simulink model "rlCOMP"  (R2024b)
settings: Solver=FixedStepAuto  StartTime=0.0  StopTime=Tf  FixedStep=0.001  RelTol=1e-3
StartFcn:
  | %scopes= find_system(bdroot,'BlockType','Scope');
  | %for i = 1:length(scopes)
  | %set_param(scopes{i},'Open','on');
  | %end
values from neighbouring files (symbols this model uses):
  amax_ego = 0.4    [MADDPG4_1.m]    (also in MADDPG4__no_rules.m; RL_COMP.m)
  amin_ego = -0.5    [MADDPG4_1.m]    (also in MADDPG4__no_rules.m; RL_COMP.m)
  Cf = 19000    [MADDPG4_1.m]    (also in MADDPG4__no_rules.m; RL_COMP.m)
  Cr = 33000    [MADDPG4_1.m]    (also in MADDPG4__no_rules.m; RL_COMP.m)
  D_default = 1.5    [MADDPG4_1.m]    (also in MADDPG4__no_rules.m; RL_COMP.m)
  e1_initial = 0    [MADDPG4_1.m]    (also in MADDPG4__no_rules.m = -0.05; RL_COMP.m = -0.05)
  e2_initial = 0.26    [MADDPG4_1.m]    (also in MADDPG4__no_rules.m = 0.05; RL_COMP.m = 0.05)
  Iz = 2875    [MADDPG4_1.m]    (also in MADDPG4__no_rules.m; RL_COMP.m)
  lf = 1.4    [MADDPG4_1.m]    (also in MADDPG4__no_rules.m; RL_COMP.m)
  lr = 1.6    [MADDPG4_1.m]    (also in MADDPG4__no_rules.m; RL_COMP.m)
  m = 1600    [MADDPG4_1.m]    (also in MADDPG4__no_rules.m; RL_COMP.m)
  t_gap = 1.4    [MADDPG4_1.m]    (also in MADDPG4__no_rules.m; RL_COMP.m)
  target = 3    [MADDPG4_1.m]    (also in MADDPG4__no_rules.m; RL_COMP.m = 1)
  tau = 0.5    [MADDPG4_1.m]    (also in MADDPG4__no_rules.m; RL_COMP.m)
  Ts = 0.1    [MADDPG4_1.m]    (also in MADDPG4__no_rules.m; RL_COMP.m)
  umax_ego = 0.2618    [MADDPG4_1.m]    (also in MADDPG4__no_rules.m; RL_COMP.m)
  umin_ego = -0.2618    [MADDPG4_1.m]    (also in MADDPG4__no_rules.m; RL_COMP.m)
  v0_FV1 = 0.5    [MADDPG4_1.m]    (also in MADDPG4__no_rules.m; RL_COMP.m)
  v0_FV2 = 0.5    [MADDPG4_1.m]    (also in MADDPG4__no_rules.m; RL_COMP.m)
  v0_LV = 0.9    [MADDPG4_1.m]    (also in MADDPG4__no_rules.m; RL_COMP.m)
  v_set = 1.5    [MADDPG4_1.m]    (also in MADDPG4__no_rules.m; RL_COMP.m)
  x0_FV1 = 1.5    [MADDPG4_1.m]    (also in MADDPG4__no_rules.m; RL_COMP.m)
  x0_FV2 = 0    [MADDPG4_1.m]    (also in MADDPG4__no_rules.m; RL_COMP.m)
  x0_LV = 3    [MADDPG4_1.m]    (also in MADDPG4__no_rules.m; RL_COMP.m)
undefined symbols (not defined in the file or in its folder): DiscIntNeverNeededParam, Speed, SteeringAngle
libraries: simulink x19, rllib x4, robotlib x4, dspfdesign x2
(part 2 of 2)

== system rlCOMP/STEER3/Subsystem1 ==
  e1 : Inport
  e2 : Inport  Port=2
  e1dot : Inport  Port=3
  e2dot : Inport  Port=4
  steer2 : Inport  Port=5
  lat2 : Inport  Port=6
  yaw2 : Inport  Port=7
  Discrete-Time Integrator : DiscreteIntegrator  SampleTime=-1  ICPrevOutput=DiscIntNeverNeededParam  ICPrevScaledInput=DiscIntNeverNeededParam
  Discrete-Time Integrator1 : DiscreteIntegrator  SampleTime=-1  ICPrevOutput=DiscIntNeverNeededParam  ICPrevScaledInput=DiscIntNeverNeededParam
  Mux : Mux  Inputs=9
  obs : Outport  VectorParamsAs1DForOutWhenUnconnected=off
  wires:
  e1/1 -> Mux/2, Discrete-Time Integrator1/1
  Mux/1 -> obs/1
  Discrete-Time Integrator1/1 -> Mux/1  "integral_error"
  e2/1 -> Mux/4, Discrete-Time Integrator/1
  Discrete-Time Integrator/1 -> Mux/3  "integral_error"
  e1dot/1 -> Mux/5
  e2dot/1 -> Mux/6
  steer2/1 -> Mux/7
  lat2/1 -> Mux/8
  yaw2/1 -> Mux/9

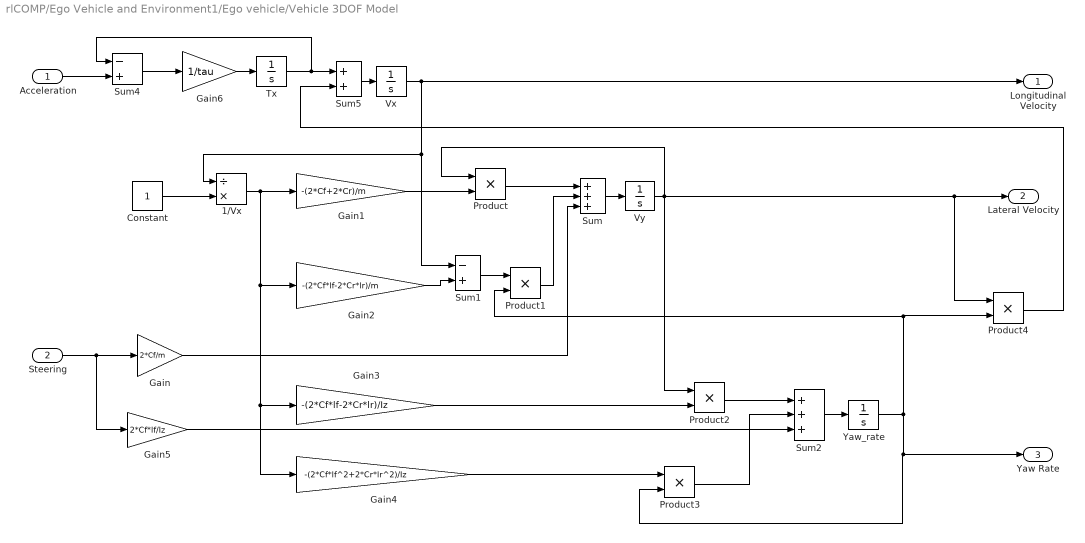
== system rlCOMP/Ego Vehicle and Environment1/Ego vehicle/Vehicle 3DOF Model ==
  Acceleration : Inport
  Steering : Inport  Port=2
  1/Vx : Product  Inputs=/*
  Constant : Constant
  Gain : Gain  Gain=2*Cf/m
  Gain1 : Gain  Gain=-(2*Cf+2*Cr)/m
  Gain2 : Gain  Gain=-(2*Cf*lf-2*Cr*lr)/m
  Gain3 : Gain  Gain=-(2*Cf*lf-2*Cr*lr)/Iz
  Gain4 : Gain  Gain=-(2*Cf*lf^2+2*Cr*lr^2)/Iz
  Gain5 : Gain  Gain=2*Cf*lf/Iz
  Gain6 : Gain  Gain=1/tau
  Product{,1..4} (5 alike) : Product
  Sum : Sum  Inputs=+++
  Sum1 : Sum  Inputs=-+
  Sum2 : Sum  Inputs=+++
  Sum4 : Sum  Inputs=-+
  Sum5 : Sum
  Tx : Integrator
  Vx : Integrator  InitialCondition=v0_FV2
  Vy : Integrator
  "Yaw_rate " : Integrator
  Longitudinal Velocity : Outport  VectorParamsAs1DForOutWhenUnconnected=off
  Lateral Velocity : Outport  Port=2  VectorParamsAs1DForOutWhenUnconnected=off
  Yaw Rate : Outport  Port=3  VectorParamsAs1DForOutWhenUnconnected=off
  wires:
  Vy/1 -> Product/1, Lateral Velocity/1, Product4/1, Product2/1
  Gain2/1 -> Sum1/2
  Product/1 -> Sum/1
  Tx/1 -> Sum5/1, Sum4/1
  Sum/1 -> Vy/1
  "Yaw_rate "/1 -> Yaw Rate/1, Product3/2, Product4/2, Product1/2
  1/Vx/1 -> Gain4/1, Gain3/1, Gain2/1, Gain1/1
  Vx/1 -> 1/Vx/1, Sum1/1, Longitudinal Velocity/1
  Product3/1 -> Sum2/2
  Steering/1 -> Gain/1, Gain5/1
  Acceleration/1 -> Sum4/2
  Sum1/1 -> Product1/1
  Gain/1 -> Sum/3
  Gain1/1 -> Product/2
  Gain6/1 -> Tx/1
  Product2/1 -> Sum2/1
  Sum5/1 -> Vx/1
  Constant/1 -> 1/Vx/2
  Product1/1 -> Sum/2
  Sum4/1 -> Gain6/1
  Gain4/1 -> Product3/1
  Product4/1 -> Sum5/2
  Gain3/1 -> Product2/2
  Gain5/1 -> Sum2/3
  Sum2/1 -> "Yaw_rate "/1

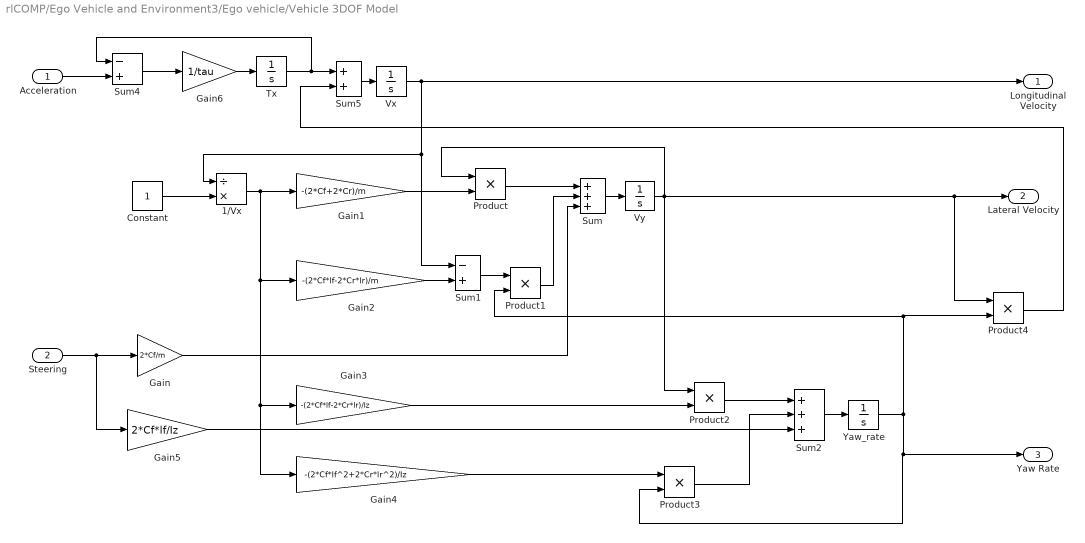
== system rlCOMP/Ego Vehicle and Environment3/Ego vehicle/Vehicle 3DOF Model ==
  Acceleration : Inport
  Steering : Inport  Port=2
  1/Vx : Product  Inputs=/*
  Constant : Constant
  Gain : Gain  Gain=2*Cf/m
  Gain1 : Gain  Gain=-(2*Cf+2*Cr)/m
  Gain2 : Gain  Gain=-(2*Cf*lf-2*Cr*lr)/m
  Gain3 : Gain  Gain=-(2*Cf*lf-2*Cr*lr)/Iz
  Gain4 : Gain  Gain=-(2*Cf*lf^2+2*Cr*lr^2)/Iz
  Gain5 : Gain  Gain=2*Cf*lf/Iz
  Gain6 : Gain  Gain=1/tau
  Product{,1..4} (5 alike) : Product
  Sum : Sum  Inputs=+++
  Sum1 : Sum  Inputs=-+
  Sum2 : Sum  Inputs=+++
  Sum4 : Sum  Inputs=-+
  Sum5 : Sum
  Tx : Integrator
  Vx : Integrator  InitialCondition=v0_FV1
  Vy : Integrator
  "Yaw_rate " : Integrator
  Longitudinal Velocity : Outport  VectorParamsAs1DForOutWhenUnconnected=off
  Lateral Velocity : Outport  Port=2  VectorParamsAs1DForOutWhenUnconnected=off
  Yaw Rate : Outport  Port=3  VectorParamsAs1DForOutWhenUnconnected=off
  wires:
  Vy/1 -> Product/1, Lateral Velocity/1, Product4/1, Product2/1
  Gain2/1 -> Sum1/2
  Product/1 -> Sum/1
  Tx/1 -> Sum5/1, Sum4/1
  Sum/1 -> Vy/1
  "Yaw_rate "/1 -> Yaw Rate/1, Product3/2, Product4/2, Product1/2
  1/Vx/1 -> Gain4/1, Gain3/1, Gain2/1, Gain1/1
  Vx/1 -> 1/Vx/1, Sum1/1, Longitudinal Velocity/1
  Product3/1 -> Sum2/2
  Steering/1 -> Gain/1, Gain5/1
  Acceleration/1 -> Sum4/2
  Sum1/1 -> Product1/1
  Gain/1 -> Sum/3
  Gain1/1 -> Product/2
  Gain6/1 -> Tx/1
  Product2/1 -> Sum2/1
  Sum5/1 -> Vx/1
  Constant/1 -> 1/Vx/2
  Product1/1 -> Sum/2
  Sum4/1 -> Gain6/1
  Gain4/1 -> Product3/1
  Product4/1 -> Sum5/2
  Gain3/1 -> Product2/2
  Gain5/1 -> Sum2/3
  Sum2/1 -> "Yaw_rate "/1

== system rlCOMP/Ego Vehicle and Environment3/Lead vehicle1/ramp1 ==
  note: 工况1：斜坡加速度
  Clock : Clock
  Constant1 : Constant  Value=20
  Constant2 : Constant  Value=40
  Ramp : simulink/Sources/Ramp  slope=0.001  start=0  InitialOutput=0
  Ramp1 : simulink/Sources/Ramp  slope=-0.001  start=20  InitialOutput=0.02
  Ramp2 : simulink/Sources/Ramp  slope=0  start=40  InitialOutput=0
  Relational Operator : RelationalOperator  Operator=<=  OutDataTypeStr=boolean  RndMeth=Simplest  InputSameDT=off
  Relational Operator1 : RelationalOperator  Operator=<=  OutDataTypeStr=boolean  RndMeth=Simplest  InputSameDT=off
  Switch : Switch  Criteria=u2 > Threshold  SaturateOnIntegerOverflow=off  InputSameDT=off
  Switch1 : Switch  Criteria=u2 > Threshold  SaturateOnIntegerOverflow=off  InputSameDT=off
  Out1 : Outport
  wires:
  Constant1/1 -> Relational Operator/2
  Ramp1/1 -> Switch1/1
  Relational Operator/1 -> Switch/2
  Switch1/1 -> Switch/3
  Relational Operator1/1 -> Switch1/2
  Clock/1 -> Relational Operator1/1, Relational Operator/1
  Ramp/1 -> Switch/1
  Constant2/1 -> Relational Operator1/2
  Ramp2/1 -> Switch1/3
  Switch/1 -> Out1/1

== system rlCOMP/Ego Vehicle and Environment3/Lead vehicle1/step1 ==
  note: 工况3：阶梯式加速-减速
  Add : Sum  Inputs=++++
  Step : Step  Time=5  After=0.2  SampleTime=0
  Step1 : Step  Time=8  After=-0.2  SampleTime=0
  Step2 : Step  Time=40  After=-0.2  SampleTime=0
  Step3 : Step  Time=43  After=0.2  SampleTime=0
  a_LV : Outport
  wires:
  Step2/1 -> Add/3
  Step3/1 -> Add/4
  Step/1 -> Add/1
  Add/1 -> a_LV/1  "a_LV"
  Step1/1 -> Add/2

== matlab function rlCOMP/MATLAB Function4 ==
  data: current_d input; is_illegal_long output; FV_v input; LV_v input; a_action input; T input; safe_d_min input
function is_illegal_long = model1(...
    current_d,FV_v, LV_v,a_action,T,safe_d_min)        
        % current_d 当前车间距 (m)
        % FV_v 跟随车速度 (m/s)
        % LV_v 引导车速度 (m/s)
        % a_action 待评估的加速度动作 (m/s²)
        % T 控制周期 (s)
        % safe_d_min 最小安全车间距 (m)

% ------------ 纵向预测模型 ------------
% 预测下一时刻车间距（考虑加速度带来的位移变化）
% 公式：Δd(k+1) = Δd(k) + (LV纵向速度 - FV纵向速度)*T + 0.5*加速度*T²
pred_d = current_d + (LV_v - FV_v) * T + 0.5 * a_action * T^2;

% ------------ 非法判定 ------------
% 若预测车间距小于安全阈值，判定为非法纵向动作
if pred_d < safe_d_min
    is_illegal_long = 1;  % 1表示非法
else
    is_illegal_long = 0;  % 0表示合法
end

% 防止车间距为负（物理意义约束）
if pred_d < 0
    pred_d = 0;
end
end

== matlab function rlCOMP/MATLAB Function5 ==
  data: current_ey input; is_illegal_lat output; FV_v input; yaw input; delta_action input; T input; L input; ey_max input
function is_illegal_lat = model2(...
    current_ey,FV_v, yaw, delta_action, T, L,ey_max) 
       % current_ey当前横向偏差 (m)
       % FV_v 跟随车速度 (m/s)
       % yaw  航向角偏差(rad)
       % delta_action 待评估的转向角动作 (rad)
       % T, L 控制周期 (s)、轴距 (m)
       % ey_max最大允许横向偏差 (m)，如±0.5m

% ------------ 横向预测模型（简化自行车模型） ------------
 % 改进1：预测下一时刻的航向角偏差（考虑转向角动作）
    % 航向角变化率 = (速度/轴距) * 转向角 → 下一时刻航向角偏差 = 当前yaw + 变化率*T
yaw_next = yaw + (FV_v / L) * delta_action * T;  % 新增：预测未来航向角偏差
% 2. 预测下一时刻横向偏差
% 公式：ey(k+1) = ey(k) + FV速度 * sin(航向角偏差) * T
pred_ey = current_ey + FV_v * sin(yaw_next) * T;

% 3. 预测航向角变化（受转向角影响）
% 公式：θ(k+1) = θ(k) + (FV速度 / 轴距) * 转向角 * T
% （注：此步用于修正后续预测，当前仅需输出横向偏差）

% ------------ 非法判定 ------------
% 若预测横向偏差超出±ey_max，判定为非法横向动作
if abs(pred_ey) > ey_max
    is_illegal_lat = 1;  % 1表示非法
else
    is_illegal_lat = 0;  % 0表示合法
end
end

== matlab function rlCOMP/MATLAB Function6 ==
  data: is_illegal_long input; a_raw input; a_output output; FV_v input; LV_v input; T input
function a_output = correction1(...
    is_illegal_long,  a_raw, FV_v, LV_v, T)        
    % 输入参数：
    %   is_illegal_long：纵向非法标志（1=非法，0=合法）
    %   a_raw：原始加速度动作 (m/s²)
    %   FV_v：跟随车当前速度 (m/s)
    %   LV_v：引导车当前速度 (m/s)
    %   T：控制周期 (s)（如0.1s，需与仿真步长一致）
    %   decel_min：最大允许减速（最激进，如-5.0m/s²，车辆物理极限）
    %   decel_max：最小允许减速（最温和，如-1.0m/s²，避免不必要的急刹）
    
    % 合法时直接输出原始动作
    if ~is_illegal_long
        a_output = a_raw;
        return;
    end
    
    % 非法时：动态计算所需减速，确保FV速度≤LV速度（阻止车间距缩小）
    % 1. 计算相对速度（FV比LV快多少）
    relative_v = FV_v - LV_v;  % >0表示FV在靠近LV
    
    if relative_v <= 0  % FV速度≤LV速度（此时车间距不会缩小，仅需轻微减速拉开距离）
        a_output = 0;  % 温和减速（如0m/s²）
        
    else  % FV速度>LV速度（必须快速减速至≤LV速度）
        % 2. 计算“刚好使FV在下一周期速度≤LV速度”所需的减速
        % 公式：FV_v + a*T ≤ LV_v → a ≤ (LV_v - FV_v)/T
        required_decel = (LV_v - FV_v) / T;  % 理论所需减速（可能很激进）
        
        % 3. 限制在车辆物理能力范围内（避免超过最大减速）
        a_output = max(required_decel, -0.5);  % 不超过最激进减速
        a_output = min(a_output, 0);        % 不低于最温和减速
    end
end

== matlab function rlCOMP/MATLAB Function7 ==
  data: is_illegal_lat input; delta_raw input; delta_output output; FV_v input; current_ey input; ey_max input; L input
function delta_output = correction2(...
    is_illegal_lat, delta_raw, FV_v, current_ey, ey_max, L) 
    % 输入参数：
    %   is_illegal_lat：横向非法标志（1=非法，0=合法）
    %   delta_raw：原始转向角动作 (rad)
    %   FV_v：跟随车速度（最高1.5m/s）(m/s)
    %   current_ey：当前横向偏差 (m)
    %   ey_max：最大允许横向偏差 (m)（如0.2m）
    %   L：轴距 (m)
    
    % 合法时直接输出原始动作
    if ~is_illegal_lat
        delta_output = delta_raw;
        return;
    end
    
    % 改进1：根据偏差超限程度动态调整衰减比例（低速下修正更激进）
    over_ratio = abs(current_ey) / ey_max;  % 超限比例（如0.3m/0.2m=1.5）
    if over_ratio <= 1.2  % 轻微超限（1.0~1.2倍阈值）
        decay_ratio = 0.6;  % 比原代码更激进（原0.7）
    elseif over_ratio <= 1.5  % 中度超限（1.2~1.5倍）
        decay_ratio = 0.4;  % 比原代码更激进（原0.5）
    else  % 严重超限（>1.5倍）
        decay_ratio = 0.2;  % 大幅加快回正（原0.3）
    end
    
    % 改进2：针对低速场景的速度适配（最高1.5m/s，无需限制回正速度）
    if FV_v < 0.5  % 极低速度（<0.5m/s，如起步/停车）
        decay_ratio = decay_ratio * 0.7;  % 进一步加快回正（低速下安全冗余高）
    elseif FV_v < 1.0  % 中低速（0.5~1.0m/s）
        decay_ratio = decay_ratio * 0.85;  % 适度加快回正
    else  % 较高速度（1.0~1.5m/s，您场景中的最高速）
        decay_ratio = decay_ratio * 1.0;  % 保持当前修正力度（无需减缓）
    end
    
    % 改进3：低速下的理想转向角计算（增强修正导向性）
    % 低速时横向偏差修正需要更大转向角（速度低，相同转向角的修正效果弱）
    % 系数从0.1提高到0.3（低速专属调整），确保快速抵消偏差
    ideal_delta = -sign(current_ey) * min(0.52, 0.3 * abs(current_ey) / (FV_v + 1e-6));
    
    % 混合修正：原始动作按比例衰减 + 理想转向角引导
    delta_output = delta_raw * decay_ratio + ideal_delta * (1 - decay_ratio);
end

== matlab function rlCOMP/Ego Vehicle and Environment1/curvature1/M-curve ==
  data: s input; rho output
function rho = fcn(s)
% 根据输入s计算输出rho
if s >= 0 && s < 5
  rho = 0;
elseif s >= 5 && s < 13
  rho = 0.1;
elseif s >= 13 && s < 25
  rho = -0.0667;
elseif s >= 25 && s < 27
  rho = 0;
elseif s >= 27 && s < 33
  rho = -0.05;
elseif s >= 33 && s < 53
  rho = 0.03;
elseif s >= 53 && s < 59
    rho = -0.05;
elseif s >= 59 && s < 61
    rho = 0;
elseif s >= 61 && s < 73
  rho = -0.0667;
elseif s >= 73 && s < 81
  rho = 0.1;
else  % s >= 70
  rho = 0;
end

== matlab function rlCOMP/Ego Vehicle and Environment1/curvature1/N-curve ==
  data: s input; rho output
function rho = fcn(s)
% 根据输入s计算输出rho
if s >= 0 && s < 5
  rho = 0;
elseif s >= 5 && s < 10
  rho = 0.025*4;
elseif s >= 10 && s < 30
  rho = -0.025;
elseif s >= 30 && s < 40
  rho = -0.0855;
elseif s >= 40 && s < 60
  rho = 0.057;
else  % s >= 60
  rho = 0;
end

== matlab function rlCOMP/Ego Vehicle and Environment1/curvature1/S-curve ==
  data: s input; rho output
function rho = fcn(s)
% 根据输入s计算输出rho
if s >= 0 && s < 10
  rho = 0;
elseif s >= 10 && s < 40
  rho = 0.005*4;
elseif s >= 40 && s < 70
  rho = -0.005*4;
else  % s >= 70
  rho = 0;
end

== matlab function rlCOMP/Ego Vehicle and Environment3/curvature1/M-curve ==
  data: s input; rho output
function rho = fcn(s)
% 根据输入s计算输出rho
if s >= 0 && s < 5
  rho = 0;
elseif s >= 5 && s < 13
  rho = 0.1;
elseif s >= 13 && s < 25
  rho = -0.0667;
elseif s >= 25 && s < 27
  rho = 0;
elseif s >= 27 && s < 33
  rho = -0.05;
elseif s >= 33 && s < 53
  rho = 0.03;
elseif s >= 53 && s < 59
    rho = -0.05;
elseif s >= 59 && s < 61
    rho = 0;
elseif s >= 61 && s < 73
  rho = -0.0667;
elseif s >= 73 && s < 81
  rho = 0.1;
else  % s >= 70
  rho = 0;
end

== matlab function rlCOMP/Ego Vehicle and Environment3/curvature1/N-curve ==
  data: s input; rho output
function rho = fcn(s)
% 根据输入s计算输出rho
if s >= 0 && s < 5
  rho = 0;
elseif s >= 5 && s < 10
  rho = 0.025*4;
elseif s >= 10 && s < 30
  rho = -0.025;
elseif s >= 30 && s < 40
  rho = -0.0855;
elseif s >= 40 && s < 60
  rho = 0.057;
else  % s >= 60
  rho = 0;
end

== matlab function rlCOMP/Ego Vehicle and Environment3/curvature1/S-curve ==
  data: s input; rho output
function rho = fcn(s)
% 根据输入s计算输出rho
if s >= 0 && s < 10
  rho = 0;
elseif s >= 10 && s < 40
  rho = 0.005*4;
elseif s >= 40 && s < 70
  rho = -0.005*4;
else  % s >= 70
  rho = 0;
end

== matlab function rlCOMP/MATLAB Function ==
  data: current_d input; is_illegal_long output; FV_v input; LV_v input; a_action input; T input; safe_d_min input
function is_illegal_long = model1(...
    current_d,FV_v, LV_v,a_action,T,safe_d_min)        
        % current_d 当前车间距 (m)
        % FV_v 跟随车速度 (m/s)
        % LV_v 引导车速度 (m/s)
        % a_action 待评估的加速度动作 (m/s²)
        % T 控制周期 (s)
        % safe_d_min 最小安全车间距 (m)

% ------------ 纵向预测模型 ------------
% 预测下一时刻车间距（考虑加速度带来的位移变化）
% 公式：Δd(k+1) = Δd(k) + (LV纵向速度 - FV纵向速度)*T + 0.5*加速度*T²
pred_d = current_d + (LV_v - FV_v) * T + 0.5 * a_action * T^2;

% ------------ 非法判定 ------------
% 若预测车间距小于安全阈值，判定为非法纵向动作
if pred_d < safe_d_min
    is_illegal_long = 1;  % 1表示非法
else
    is_illegal_long = 0;  % 0表示合法
end

% 防止车间距为负（物理意义约束）
if pred_d < 0
    pred_d = 0;
end
end

== matlab function rlCOMP/MATLAB Function1 ==
  data: current_ey input; is_illegal_lat output; FV_v input; yaw input; delta_action input; T input; L input; ey_max input
function is_illegal_lat = model2(...
    current_ey,FV_v, yaw, delta_action, T, L,ey_max) 
       % current_ey当前横向偏差 (m)
       % FV_v 跟随车速度 (m/s)
       % yaw  航向角偏差(rad)
       % delta_action 待评估的转向角动作 (rad)
       % T, L 控制周期 (s)、轴距 (m)
       % ey_max最大允许横向偏差 (m)，如±0.5m

% ------------ 横向预测模型（简化自行车模型） ------------
 % 改进1：预测下一时刻的航向角偏差（考虑转向角动作）
    % 航向角变化率 = (速度/轴距) * 转向角 → 下一时刻航向角偏差 = 当前yaw + 变化率*T
yaw_next = yaw + (FV_v / L) * delta_action * T;  % 新增：预测未来航向角偏差
% 2. 预测下一时刻横向偏差
% 公式：ey(k+1) = ey(k) + FV速度 * sin(航向角偏差) * T
pred_ey = current_ey + FV_v * sin(yaw_next) * T;

% 3. 预测航向角变化（受转向角影响）
% 公式：θ(k+1) = θ(k) + (FV速度 / 轴距) * 转向角 * T
% （注：此步用于修正后续预测，当前仅需输出横向偏差）

% ------------ 非法判定 ------------
% 若预测横向偏差超出±ey_max，判定为非法横向动作
if abs(pred_ey) > ey_max
    is_illegal_lat = 1;  % 1表示非法
else
    is_illegal_lat = 0;  % 0表示合法
end
end

== matlab function rlCOMP/MATLAB Function2 ==
  data: is_illegal_long input; a_raw input; a_output output; FV_v input; LV_v input; T input
function a_output = correction1(...
    is_illegal_long,  a_raw, FV_v, LV_v, T)        
    % 输入参数：
    %   is_illegal_long：纵向非法标志（1=非法，0=合法）
    %   a_raw：原始加速度动作 (m/s²)
    %   FV_v：跟随车当前速度 (m/s)
    %   LV_v：引导车当前速度 (m/s)
    %   T：控制周期 (s)（如0.1s，需与仿真步长一致）
    %   decel_min：最大允许减速（最激进，如-5.0m/s²，车辆物理极限）
    %   decel_max：最小允许减速（最温和，如-1.0m/s²，避免不必要的急刹）
    
    % 合法时直接输出原始动作
    if ~is_illegal_long
        a_output = a_raw;
        return;
    end
    
    % 非法时：动态计算所需减速，确保FV速度≤LV速度（阻止车间距缩小）
    % 1. 计算相对速度（FV比LV快多少）
    relative_v = FV_v - LV_v;  % >0表示FV在靠近LV
    
    if relative_v <= 0  % FV速度≤LV速度（此时车间距不会缩小，仅需轻微减速拉开距离）
        a_output = 0;  % 温和减速（如0m/s²）
        
    else  % FV速度>LV速度（必须快速减速至≤LV速度）
        % 2. 计算“刚好使FV在下一周期速度≤LV速度”所需的减速
        % 公式：FV_v + a*T ≤ LV_v → a ≤ (LV_v - FV_v)/T
        required_decel = (LV_v - FV_v) / T;  % 理论所需减速（可能很激进）
        
        % 3. 限制在车辆物理能力范围内（避免超过最大减速）
        a_output = max(required_decel, -0.5);  % 不超过最激进减速
        a_output = min(a_output, 0);        % 不低于最温和减速
    end
end

== matlab function rlCOMP/MATLAB Function3 ==
  data: is_illegal_lat input; delta_raw input; delta_output output; FV_v input; current_ey input; ey_max input; L input
function delta_output = correction2(...
    is_illegal_lat, delta_raw, FV_v, current_ey, ey_max, L) 
    % 输入参数：
    %   is_illegal_lat：横向非法标志（1=非法，0=合法）
    %   delta_raw：原始转向角动作 (rad)
    %   FV_v：跟随车速度（最高1.5m/s）(m/s)
    %   current_ey：当前横向偏差 (m)
    %   ey_max：最大允许横向偏差 (m)（如0.2m）
    %   L：轴距 (m)
    
    % 合法时直接输出原始动作
    if ~is_illegal_lat
        delta_output = delta_raw;
        return;
    end
    
    % 改进1：根据偏差超限程度动态调整衰减比例（低速下修正更激进）
    over_ratio = abs(current_ey) / ey_max;  % 超限比例（如0.3m/0.2m=1.5）
    if over_ratio <= 1.2  % 轻微超限（1.0~1.2倍阈值）
        decay_ratio = 0.6;  % 比原代码更激进（原0.7）
    elseif over_ratio <= 1.5  % 中度超限（1.2~1.5倍）
        decay_ratio = 0.4;  % 比原代码更激进（原0.5）
    else  % 严重超限（>1.5倍）
        decay_ratio = 0.2;  % 大幅加快回正（原0.3）
    end
    
    % 改进2：针对低速场景的速度适配（最高1.5m/s，无需限制回正速度）
    if FV_v < 0.5  % 极低速度（<0.5m/s，如起步/停车）
        decay_ratio = decay_ratio * 0.7;  % 进一步加快回正（低速下安全冗余高）
    elseif FV_v < 1.0  % 中低速（0.5~1.0m/s）
        decay_ratio = decay_ratio * 0.85;  % 适度加快回正
    else  % 较高速度（1.0~1.5m/s，您场景中的最高速）
        decay_ratio = decay_ratio * 1.0;  % 保持当前修正力度（无需减缓）
    end
    
    % 改进3：低速下的理想转向角计算（增强修正导向性）
    % 低速时横向偏差修正需要更大转向角（速度低，相同转向角的修正效果弱）
    % 系数从0.1提高到0.3（低速专属调整），确保快速抵消偏差
    ideal_delta = -sign(current_ey) * min(0.52, 0.3 * abs(current_ey) / (FV_v + 1e-6));
    
    % 混合修正：原始动作按比例衰减 + 理想转向角引导
    delta_output = delta_raw * decay_ratio + ideal_delta * (1 - decay_ratio);
end
